simulink model "simulink_test"  (R2023a)
settings: Solver=VariableStepAuto  StartTime=0.0  StopTime=15.05  RelTol=1e-3
undefined symbols (not defined in the file or in its folder): cb, cqt, g, J1, J2, J3, l, m, sb
settings Model: Creator=m_ara  LastModifiedBy=m_ara

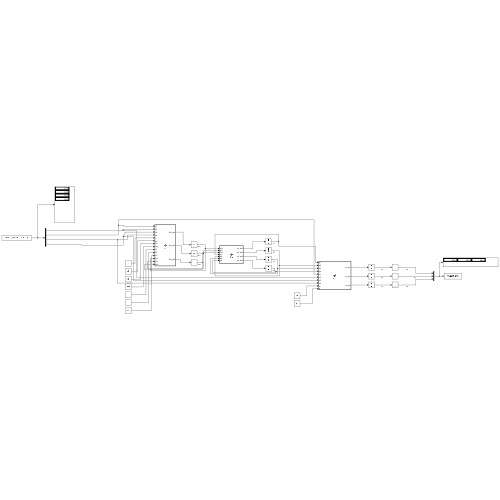
[thumbnail: Simulink's stored preview of the top-level diagram]
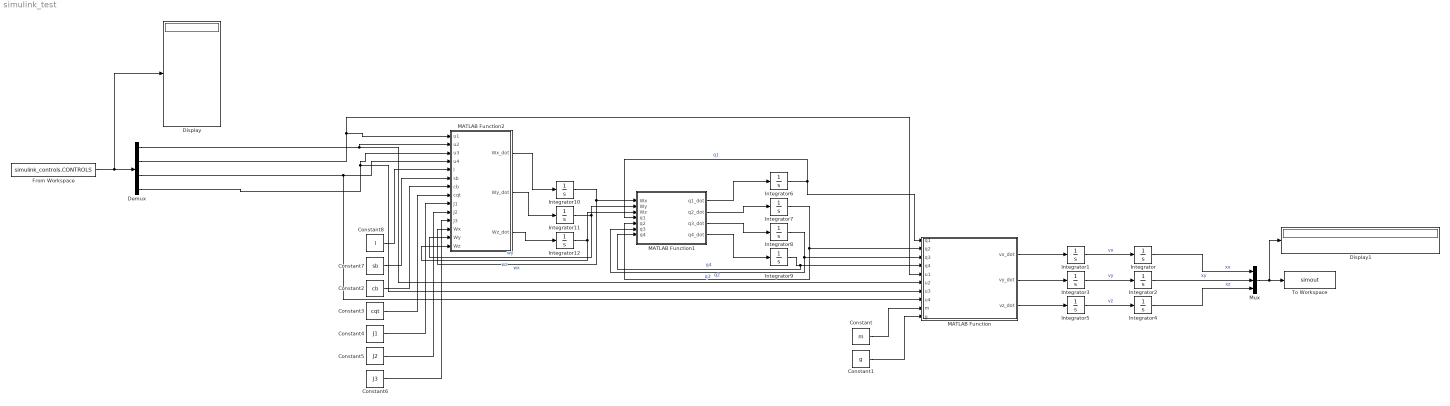
== system simulink_test ==
  Constant : Constant  Value=m
  Constant1 : Constant  Value=g
  Constant2 : Constant  Value=cb
  Constant3 : Constant  Value=cqt
  Constant4 : Constant  Value=J1
  Constant5 : Constant  Value=J2
  Constant6 : Constant  Value=J3
  Constant7 : Constant  Value=sb
  Constant8 : Constant  Value=l
  Demux : Demux
  Display : Display
      settings: Decimation=4
  Display1 : Display
  From Workspace : FromWorkspace  VariableName=simulink_controls.CONTROLS  OutDataTypeStr=double  SampleTime=0.005
  Integrator{,1..5,7..12} (12 alike) : Integrator
  Integrator6 : Integrator  InitialCondition=1
  MATLAB Function : MATLAB Function  TreatAsAtomicUnit=on
  MATLAB Function1 : MATLAB Function  TreatAsAtomicUnit=on
  MATLAB Function2 : MATLAB Function  TreatAsAtomicUnit=on
  Mux : Mux  Inputs=3
  To Workspace : ToWorkspace  VariableName=simout  SaveFormat=Timeseries  SampleTime=-1
  wires:
  Integrator/1 -> Mux/1  "xx"
  Integrator1/1 -> Integrator/1  "vx"
  MATLAB Function/1(vx_dot) -> Integrator1/1
  MATLAB Function/2(vy_dot) -> Integrator3/1
  MATLAB Function/3(vz_dot) -> Integrator5/1
  Integrator3/1 -> Integrator2/1  "vy"
  Integrator5/1 -> Integrator4/1  "vz"
  Integrator2/1 -> Mux/2  "xy"
  Integrator4/1 -> Mux/3  "xz"
  Mux/1 -> Display1/1, To Workspace/1
  Constant/1 -> MATLAB Function/9(m)
  Constant1/1 -> MATLAB Function/10(g)
  Integrator6/1 -> MATLAB Function1/4(q1), MATLAB Function/1(q1)  "q1"
  Integrator7/1 -> MATLAB Function1/5(q2), MATLAB Function/2(q2)  "q2"
  Integrator8/1 -> MATLAB Function1/6(q3), MATLAB Function/3(q3)  "q3"
  Integrator9/1 -> MATLAB Function1/7(q4), MATLAB Function/4(q4)  "q4"
  MATLAB Function1/1(q1_dot) -> Integrator6/1
  MATLAB Function1/2(q2_dot) -> Integrator7/1
  MATLAB Function1/3(q3_dot) -> Integrator8/1
  MATLAB Function1/4(q4_dot) -> Integrator9/1
  Integrator10/1 -> MATLAB Function2/12(Wx), MATLAB Function1/1(Wx)  "wx"
  Integrator11/1 -> MATLAB Function2/13(Wy), MATLAB Function1/2(Wy)  "wy"
  Integrator12/1 -> MATLAB Function2/14(Wz), MATLAB Function1/3(Wz)  "wz"
  MATLAB Function2/2(Wy_dot) -> Integrator11/1
  MATLAB Function2/3(Wz_dot) -> Integrator12/1
  MATLAB Function2/1(Wx_dot) -> Integrator10/1
  Constant8/1 -> MATLAB Function2/5(l)
  Constant7/1 -> MATLAB Function2/6(sb)
  Constant2/1 -> MATLAB Function2/7(cb)
  Constant3/1 -> MATLAB Function2/8(cqt)
  Constant4/1 -> MATLAB Function2/9(J1)
  Constant5/1 -> MATLAB Function2/10(J2)
  Constant6/1 -> MATLAB Function2/11(J3)
  Demux/2 -> MATLAB Function/5(u1), MATLAB Function2/1(u1)
  Demux/1 -> MATLAB Function/6(u2), MATLAB Function2/2(u2)
  Demux/4 -> MATLAB Function2/3(u3), MATLAB Function/7(u3)
  Demux/3 -> MATLAB Function/8(u4), MATLAB Function2/4(u4)
  From Workspace/1 -> Display/1, Demux/1

== matlab function simulink_test/MATLAB Function1 ==
  data: Wx input; q1_dot output; Wy input; Wz input; q2_dot output; q3_dot output; q4_dot output; q1 input; q2 input; q3 input; q4 input
function [q1_dot,q2_dot,q3_dot,q4_dot] = fcn(Wx,Wy,Wz,q1,q2,q3,q4)

q1_dot = -0.5*q2*Wx - 0.5*q3*Wy - 0.5*q4*Wz;
q2_dot = 0.5*q1*Wx - 0.5*q4*Wy + 0.5*q3*Wz;
q3_dot = 0.5*q4*Wx + 0.5*q1*Wy - 0.5*q2*Wz;
q4_dot = 0.5*q2*Wy - 0.5*q3*Wx + 0.5*q1*Wz;

end

== matlab function simulink_test/MATLAB Function ==
  data: q1 input; vx_dot output; q2 input; q3 input; q4 input; u1 input; u2 input; u3 input; u4 input; m input; vy_dot output; vz_dot output; g input
function [vx_dot,vy_dot,vz_dot]= fcn(q1,q2,q3,q4,u1,u2,u3,u4,m,g)


% Acceleration 
vx_dot = -(((2*q1*q3 + 2*q2*q4)*(u1 + u2 + u3 + u4))/m);
vy_dot = (((2*q1*q2 - 2*q3*q4)*(u1 + u2 + u3 + u4))/m);
vz_dot = g - (((2*q1*q1 + 2*q4*q4 - 1)*(u1 + u2 + u3 + u4))/m);


end

== matlab function simulink_test/MATLAB Function2 ==
  data: u1 input; Wx_dot output; u2 input; u3 input; u4 input; l input; sb input; cb input; cqt input; J1 input; J2 input; J3 input; Wy_dot output; Wz_dot output; Wx input; Wy input; Wz input
function [Wx_dot,Wy_dot,Wz_dot]= fcn(u1,u2,u3,u4,l,sb,cb,cqt,J1,J2,J3,Wx,Wy,Wz)

Wx_dot = -(l*sb*u1 - l*sb*u2 - l*sb*u3 + l*sb*u4 - J2*Wy*Wz + J3*Wy*Wz)/J1;
Wy_dot = (l*cb*u1 - l*cb*u2 + l*cb*u3 - l*cb*u4 - J1*Wx*Wz + J3*Wx*Wz)/J2;
Wz_dot = (cqt*u1 + cqt*u2 - cqt*u3 - cqt*u4 + J1*Wx*Wy - J2*Wx*Wy)/J3;

end
